simulink model "LQR_Controller"  (R2018a)
settings: Solver=VariableStepAuto  StartTime=0.0  StopTime=5  MaxStep=1e-3  RelTol=1e-3
values from neighbouring files (symbols this model uses):
  A = [0 1;1000 0]    [Parameters.m]
  B = [0;20]    [Parameters.m]
  C = [1 0]    [Parameters.m]
  L = Lt'    [Parameters.m]
  N = 1/dcgain(ss(A-B*K,B,C,D))    [Parameters.m]
undefined symbols (not defined in the file or in its folder): K
settings Model: Creator=Usuario  LastModifiedBy=Usuario

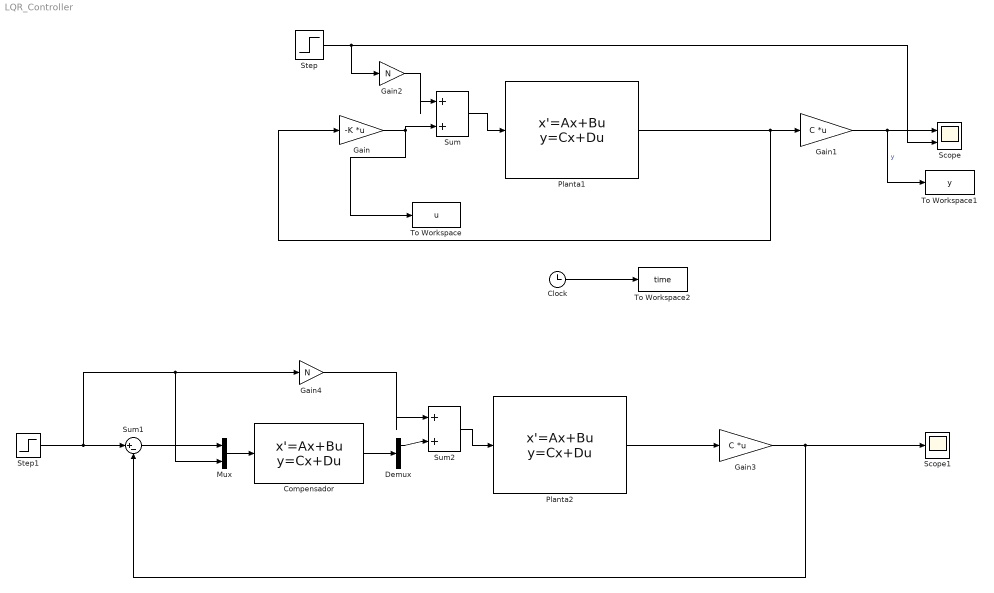
== system LQR_Controller ==
  Clock : Clock
  Compensador : StateSpace  A=A-B*K-L*C  B=[-L B*N+L]  C=[-K;0 0]  D=zeros(2,2)  InitialCondition=0
  Demux : Demux  Outputs=2
  Gain : Gain  Gain=-K  Multiplication=Matrix(K*u) (u vector)
  Gain1 : Gain  Gain=C  Multiplication=Matrix(K*u) (u vector)
  Gain2 : Gain  Gain=N
  Gain3 : Gain  Gain=C  Multiplication=Matrix(K*u) (u vector)
  Gain4 : Gain  Gain=N
  Mux : Mux  Inputs=2
  Planta1 : StateSpace  A=A  B=B  C=eye(2)  D=zeros(2,1)  InitialCondition=[0.1 0.1]
  Planta2 : StateSpace  A=A  B=B  C=eye(2)  D=zeros(2,1)  InitialCondition=[0.1 0.1]
  Scope : Scope  NumInputPorts=2
  Scope1 : Scope
  Step : Step  SampleTime=0
  Step1 : Step  SampleTime=0
  Sum : Sum  Inputs=|++
  Sum1 : Sum  Inputs=|+-
  Sum2 : Sum  Inputs=|++
  To Workspace : ToWorkspace  VariableName=u  SampleTime=-1
      settings: Save2DSignal=2-D array (concatenate along first dimension)
  To Workspace1 : ToWorkspace  VariableName=y  SampleTime=-1
      settings: Save2DSignal=2-D array (concatenate along first dimension)
  To Workspace2 : ToWorkspace  VariableName=time  SampleTime=-1
      settings: Save2DSignal=2-D array (concatenate along first dimension)
  wires:
  Planta1/1 -> Gain1/1, Gain/1
  Gain1/1 -> To Workspace1/1, Scope/1  "y"
  Gain/1 -> Sum/2, To Workspace/1
  Clock/1 -> To Workspace2/1
  Sum/1 -> Planta1/1
  Gain2/1 -> Sum/1
  Step/1 -> Scope/2, Gain2/1
  Planta2/1 -> Gain3/1
  Gain3/1 -> Scope1/1, Sum1/2
  Step1/1 -> Sum1/1, Mux/2, Gain4/1
  Sum2/1 -> Planta2/1
  Gain4/1 -> Sum2/1
  Sum1/1 -> Mux/1
  Mux/1 -> Compensador/1
  Compensador/1 -> Demux/1
  Demux/1 -> Sum2/2
